simulink model "ProgettoFinaleFSR"  (R2024a)
settings: Solver=VariableStepAuto  StartTime=0.0  StopTime=30  RelTol=1e-3
PreLoadFcn:
  | Ts = 1e-3;
  | m = 1;
InitFcn:
  | %% INITIALIZATION
  | main
  | 
  | %% UAV PARAMETERS
  | 
  | %% SAMPLING TIME
  | Ts=0.001;
  | 
  | %% PLANNER
  | % t_iniz = 0;
  | % ttot=20; %duration
  | % tdead=10; %dead time to evaluate the steady-state
  | % tot_time = ttot + tdead;
  | % t1=linspace(0,ttot,round(ttot/Ts));
  | % t=linspace(0,ttot+tdead,round(ttot/Ts)+round(tdead/Ts));
  | % p= zeros(4,length(t1)); dot_p= zeros(4,length(t1)); ddot_p= zeros(4,length(t1));
  | % p_d= zeros(4,length(t)); dot_p_d= zeros(4,length(t)); ddot_p_d= zeros(4,length(t));
  | % %Initial and final conditions
  | % x0= 0; xf=1; dot_x0= 0; dot_xf=0; ddot_x0=0; ddot_xf=0; dddot_x0 = 0; dddot_xf = 0;
  | % y0= 0; yf=1; dot_y0= 0; dot_yf=0; ddot_y0=0; ddot_yf=0; dddot_y0 = 0; dddot_yf = 0;
  | % z0= -1; zf=-4; dot_z0= 0; dot_zf=0; ddot_z0=0; ddot_zf=0; dddot_z0 = 0; dddot_zf = 0;
  | % psi0 = 0;
  | % psif=deg2rad(20); dot_psi0= 0; dot_psif=0; ddot_psi0=0; ddot_psif=0; dddot_psi0 = 0; dddot_psif = 0;
  | % p0=[x0,y0,z0,psi0]; dot_p0=[dot_x0,dot_y0,dot_z0,dot_psi0]; ddot_p0=[ddot_x0,ddot_y0,ddot_z0,ddot_psi0]; dddot_p0=[dddot_x0,dddot_y0,dddot_z0,dddot_psi0];
  | % pf=[xf,yf,zf,psif]; dot_pf=[dot_xf,dot_yf,dot_zf,dot_psif]; ddot_pf=[ddot_xf,ddot_yf,ddot_zf,ddot_psif]; dddot_pf=[dddot_xf,dddot_yf,dddot_zf,dddot_psif];
  | % %5-th order polynomial
  | % a0=zeros(1,4); a1=zeros(1,4); a2=zeros(1,4); a3=zeros(1,4); a4=zeros(1,4); a5=zeros(1,4); a6 = zeros(1,4); a7 = zeros(1,4);
  | %
  | % for j=1:4
  | %     A = [t_iniz^7, t_iniz^6, t_iniz^5, t_iniz^4, t_iniz^3, t_iniz^2, t_iniz, 1;
  | %         ttot^7, ttot^6, ttot^5, ttot^4, ttot^3, ttot^2, ttot, 1;
  | %         7*t_iniz^6, 6*t_iniz^5, 5*t_iniz^4, 4*t_iniz^3, 3*t_iniz^2, 2*t_iniz, 1, 0;
  | %         7*ttot^6, 6*ttot^5, 5*ttot^4, 4*ttot^3, 3*ttot^2, 2*ttot, 1, 0;
  | %         42*t_iniz^5, 30*t_iniz^4, 20*t_iniz^3, 12*t_iniz^2, 6*t_iniz, 2, 0, 0;
  | %         42*ttot^5, 30*ttot^4, 20*ttot^3, 12*ttot^2, 6*ttot, 2, 0, 0;
  | %         210*t_iniz^4, 120*t_iniz^3, 60*t_iniz^2, 24*t_iniz, 6, 0, 0, 0;
  | %         210*ttot^4, 120*ttot^3, 60*ttot^2, 24*ttot, 6, 0, 0, 0];
  | %     b = [p0(j) pf(j) dot_p0(j) dot_pf(j) ddot_p0(j) ddot_pf(j) dddot_p0(j) dddot_pf(j)]';
  | %     a_temp = A\b;
  | %     a7(j) = a_temp(1);
  | %     a6(j) = a_temp(2);
  | %     a5(j) = a_temp(3);
  | %     a4(j) = a_temp(4);
  | %     a3(j) = a_temp(5);
  | %     a2(j) = a_temp(6);
  | %     a1(j) = a_temp(7);
  | %     a0(j) = a_temp(8);
  | %
  | %     %trajectories
  | %     p(j,:)=a7(j)*t1.^7 + a6(j)*t1.^6 + a5(j)*t1.^5 +a4(j)*t1.^4 +a3(j)*t1.^3 +a2(j)*t1.^2 +a1(j)*t1 +a0(j);
  | %     dot_p(j,:) = 7*a7(j)*t1.^6 + 6*a6(j)*t1.^5 + 5*a5(j)*t1.^4 +4*a4(j)*t1.^3 +3*a3(j)*t1.^2 +2*a2(j)*t1 +a1(j);
  | %     ddot_p(j,:) = 42*a7(j)*t1.^5 + 30*a6(j)*t1.^4 + 5*4*a5(j)*t1.^3 +4*3*a4(j)*t1.^2 +3*2*a3(j)*t1 +2*a2(j);
  | %     %addition of the stead-state terms
  | %     p_d(j,:)=[p(j,:) zeros(1,round(tdead/Ts))+pf(j)];
  | %     dot_p_d(j,:)=[dot_p(j,:) zeros(1,round(tdead/Ts))+dot_pf(j)];
  | %     ddot_p_d(j,:)=[ddot_p(j,:) zeros(1,round(tdead/Ts))+ddot_pf(j)];
  | % end
  | % %data for Simulink
  | % pos_0 = [x0 y0 z0];
  | % lin_vel_0 = [dot_x0 dot_y0 dot_z0];
  | % w_bb_0 = [0 0 0];
  | % csi_d=p_d(1:3,:); dot_csi_d=dot_p_d(1:3,:); ddot_csi_d=ddot_p_d(1:3,:);
  | % psi_d=p_d(4,:); dot_psi_d=dot_p_d(4,:); ddot_psi_d=ddot_p_d(4,:);
values from neighbouring files (symbols this model uses):
  g = 9.81    [main.m]
  intv = [intv,v(i).vec]    [main.m]
  k = ones(r,1)    [gainvalue.m]    (also in main.m = gainvalue(r,a(2:end)))
settings Model: Creator=fabioruggiero  LastModifiedBy=Luca
settings ModelReferenceCC: EnableRefExpFcnMdlSchedulingChecks=on
settings RTWCC: GPUComputeCapability=3.5

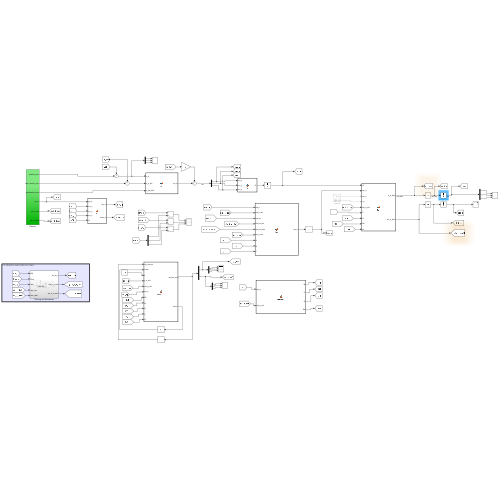
[thumbnail: Simulink's stored preview of the top-level diagram]
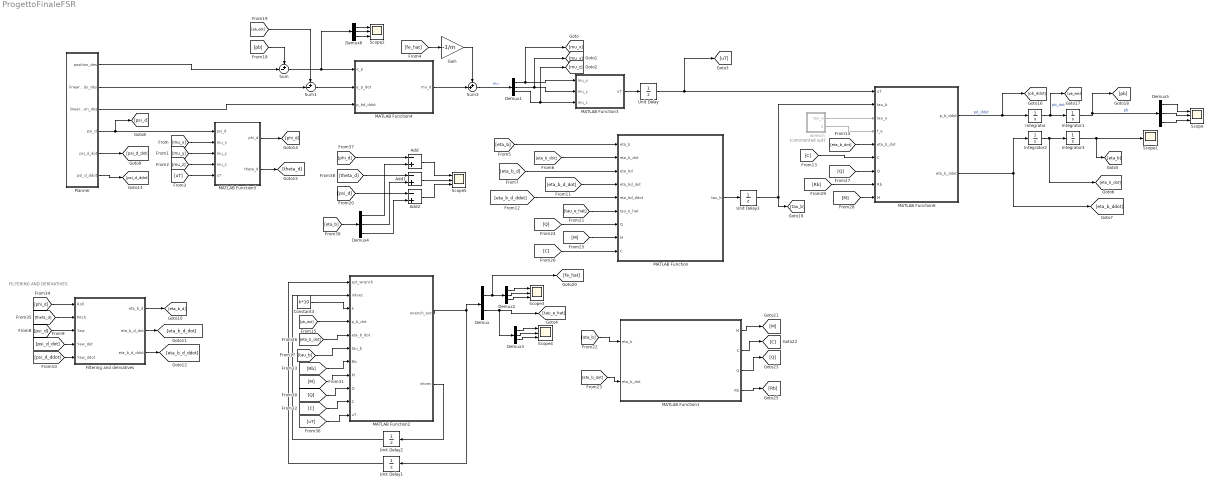
== system ProgettoFinaleFSR ==
  note: FILTERING AND DERIVATIVES
  " wrench" : Subsystem  Commented=on
  Add : Sum  Inputs=-+
  Add1 : Sum  Inputs=-+
  Add2 : Sum  Inputs=-+
  Constant3 : Constant  Value=k*10
  Demux : Demux  Outputs=2
  Demux{1..6} (6 alike) : Demux  Outputs=3
  Filtering and derivatives : Subsystem
  Gain : Gain  Gain=-1/m
  Integrator : Integrator
  Integrator1 : Integrator  InitialCondition=[0; 0; -1]
  Integrator2 : Integrator
  Integrator3 : Integrator
  MATLAB Function : MATLAB Function  TreatAsAtomicUnit=on
  MATLAB Function1 : MATLAB Function  TreatAsAtomicUnit=on
  MATLAB Function2 : MATLAB Function  TreatAsAtomicUnit=on
  MATLAB Function3 : MATLAB Function  TreatAsAtomicUnit=on
  MATLAB Function4 : MATLAB Function  TreatAsAtomicUnit=on
  MATLAB Function5 : MATLAB Function  TreatAsAtomicUnit=on
  MATLAB Function6 : MATLAB Function  TreatAsAtomicUnit=on
  Planner : Subsystem
  Scope{,2..5} (5 alike) : Scope  NumInputPorts=3
  Scope1 : Scope
  Sum : Sum  Inputs=+-|
  Sum1 : Sum  Inputs=+-|
  Sum3 : Sum  Inputs=++|
  Unit Delay : UnitDelay  InitialCondition=m*g  SampleTime=Ts  HasFrameUpgradeWarning=on
  Unit Delay1 : UnitDelay  InitialCondition=zeros(6,1)  SampleTime=Ts  HasFrameUpgradeWarning=on
  Unit Delay2 : UnitDelay  InitialCondition=intv  SampleTime=Ts  HasFrameUpgradeWarning=on
  Unit Delay3 : UnitDelay  SampleTime=Ts  HasFrameUpgradeWarning=on
  wires:
  Planner/2(linear_velocity_des) -> Sum1/2
  MATLAB Function2/2(intvec) -> Unit Delay2/1
  Unit Delay1/1 -> MATLAB Function2/1(est_wrench)
  Constant3/1 -> MATLAB Function2/3(k)
  Unit Delay2/1 -> MATLAB Function2/2("intvec ")
  MATLAB Function2/1(wrench_ext) -> Demux/1, Unit Delay1/1
  Demux1/1 -> [mu_x], MATLAB Function3/1(mu_x)
  Demux1/2 -> [mu_y], MATLAB Function3/2(mu_y)
  Demux1/3 -> [mu_z], MATLAB Function3/3(mu_z)
  Sum/1 -> Demux6/1, MATLAB Function4/1(e_p)
  Integrator1/1 -> Demux5/1, [pb]  "pb"
  Integrator/1 -> [pb_dot], Integrator1/1  "pb_dot"
  MATLAB Function6/1(p_b_ddot) -> [pb_ddot], Integrator/1  "pd_ddot"
  Sum1/1 -> MATLAB Function4/2(e_p_dot)
  Planner/1(position_des) -> Sum/2
  Planner/4(psi_d) -> [psi_d], MATLAB Function5/1(psi_d)
  MATLAB Function5/1(phi_d) -> [phi_d]
  MATLAB Function5/2(theta_d) -> [theta_d]
  [mu_x] -> MATLAB Function5/2(mu_x)
  [mu_y] -> MATLAB Function5/3(mu_y)
  [mu_z] -> MATLAB Function5/4(mu_z)
  [uT] -> MATLAB Function5/5(uT)
  Sum3/1 -> Demux1/1  "mu"
  MATLAB Function4/1(mu_d) -> Sum3/2
  [fe_hat] -> Gain/1
  Integrator2/1 -> [eta_b_dot], Integrator3/1
  Integrator3/1 -> Scope1/1, [eta_b]
  [eta_b] -> MATLAB Function/1(eta_b)
  [eta_b_dot] -> MATLAB Function/2(eta_b_dot)
  [psi_d] -> Filtering and derivatives/3(Yaw)
  [psi_d_ddot] -> Filtering and derivatives/5(Yaw_ddot)
  [theta_d] -> Filtering and derivatives/2(Pitch)
  [phi_d] -> Filtering and derivatives/1(Roll)
  Filtering and derivatives/3(eta_b_d_ddot) -> [eta_b_d_ddot]
  Filtering and derivatives/1(eta_b_d) -> [eta_b_d]
  [psi_d_dot] -> Filtering and derivatives/4(Yaw_dot)
  Filtering and derivatives/2(eta_b_d_dot) -> [eta_b_d_dot]
  Planner/5(psi_d_dot) -> [psi_d_dot]
  Planner/6(psi_d_ddot) -> [psi_d_ddot]
  [eta_b_d] -> MATLAB Function/3(eta_bd)
  [eta_b_d_dot] -> MATLAB Function/4(eta_bd_dot)
  [eta_b_d_ddot] -> MATLAB Function/5(eta_bd_ddot)
  [C] -> MATLAB Function6/6(C)
  [eta_b_dot] -> MATLAB Function6/5(eta_b_dot)
  [eta_b_dot] -> MATLAB Function2/5(eta_b_dot)
  [tau_b] -> MATLAB Function2/6(tau_b)
  [pb] -> Sum/1
  [pb_dot] -> Sum1/1
  Planner/3(linear_acceleration_des) -> MATLAB Function4/3(p_bd_ddot)
  [tau_e_hat] -> MATLAB Function/6(tau_e_hat)
  " wrench"/1(tau_e) -> MATLAB Function6/3(tau_e)
  " wrench"/2(fe_hat) -> MATLAB Function6/4(f_e)
  [eta_b] -> MATLAB Function1/1(eta_b)
  [eta_b_dot] -> MATLAB Function1/2(eta_b_dot)
  MATLAB Function1/1(M) -> [M]
  MATLAB Function1/2(C) -> [C]
  MATLAB Function1/3(Q) -> [Q]
  MATLAB Function1/4(Rb) -> [Rb]
  [Q] -> MATLAB Function/7(Q)
  [M] -> MATLAB Function/8(M)
  [C] -> MATLAB Function/9(C)
  [Q] -> MATLAB Function6/7(Q)
  [M] -> MATLAB Function6/9(M)
  [Rb] -> MATLAB Function6/8(Rb)
  [C] -> MATLAB Function2/10(C)
  [M] -> MATLAB Function2/8(M)
  [Q] -> MATLAB Function2/9(Q)
  [Rb] -> MATLAB Function2/7(Rb)
  [uT] -> MATLAB Function2/11(uT)
  [pb_dot] -> MATLAB Function2/4(p_b_dot)
  MATLAB Function6/2(eta_b_ddot) -> [eta_b_ddot], Integrator2/1
  MATLAB Function3/1(uT) -> Unit Delay/1
  MATLAB Function/1(tau_b) -> Unit Delay3/1
  Unit Delay/1 -> [uT], MATLAB Function6/1(uT)
  Unit Delay3/1 -> MATLAB Function6/2(tau_b), [tau_b]
  Demux2/1 -> Scope3/1
  Demux2/2 -> Scope3/2
  Demux2/3 -> Scope3/3
  Demux/1 -> [fe_hat], Demux2/1
  Demux/2 -> Demux3/1, [tau_e_hat]
  Demux3/3 -> Scope4/3
  Demux3/2 -> Scope4/2
  Demux3/1 -> Scope4/1
  [eta_b] -> Demux4/1
  Add/1 -> Scope5/1
  Add1/1 -> Scope5/2
  Add2/1 -> Scope5/3
  [theta_d] -> Add1/1
  [psi_d] -> Add2/1
  [phi_d] -> Add/1
  Demux4/1 -> Add/2
  Demux4/2 -> Add1/2
  Demux4/3 -> Add2/2
  Demux5/1 -> Scope/1
  Demux5/2 -> Scope/2
  Demux5/3 -> Scope/3
  Demux6/1 -> Scope2/1
  Demux6/2 -> Scope2/2
  Demux6/3 -> Scope2/3
  Gain/1 -> Sum3/1

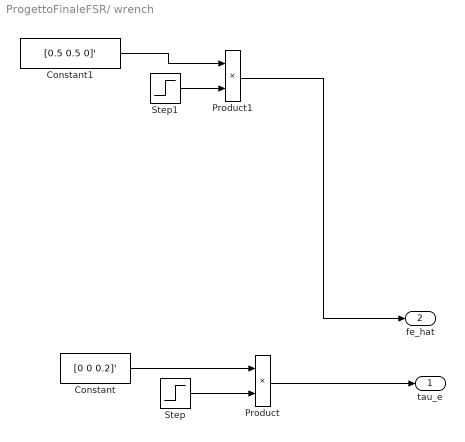
== system ProgettoFinaleFSR/ wrench ==
  Constant : Constant  Value=[0 0 0.2]'
  Constant1 : Constant  Value=[0.5 0.5 0]'
  Product : Product
  Product1 : Product
  Step : Step  Time=10  SampleTime=0
  Step1 : Step  Time=10  SampleTime=0
  tau_e : Outport
  fe_hat : Outport  Port=2
  wires:
  Step1/1 -> Product1/2
  Product/1 -> tau_e/1
  Constant1/1 -> Product1/1
  Constant/1 -> Product/1
  Step/1 -> Product/2
  Product1/1 -> fe_hat/1

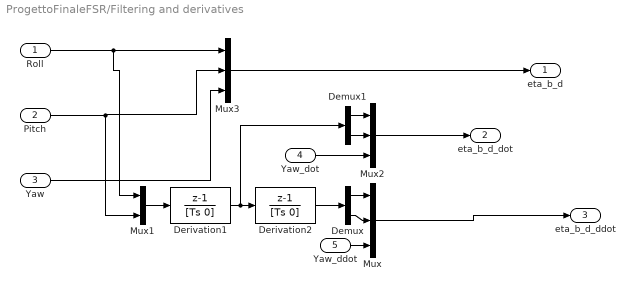
== system ProgettoFinaleFSR/Filtering and derivatives ==
  Roll : Inport
  Pitch : Inport  Port=2
  Yaw : Inport  Port=3
  Yaw_dot : Inport  Port=4
  Yaw_ddot : Inport  Port=5
  Demux : Demux  Outputs=2
  Demux1 : Demux  Outputs=2
  Derivation1 : DiscreteTransferFcn  Numerator=[1 -1]  Denominator=[Ts 0]  InitialStates=[0 0]  SampleTime=Ts
  Derivation2 : DiscreteTransferFcn  Numerator=[1 -1]  Denominator=[Ts 0]  InitialStates=[0 0]  SampleTime=Ts
  Mux : Mux  Inputs=3
  Mux1 : Mux  Inputs=2
  Mux2 : Mux  Inputs=3
  Mux3 : Mux  Inputs=3
  eta_b_d : Outport
  eta_b_d_dot : Outport  Port=2
  eta_b_d_ddot : Outport  Port=3
  wires:
  Derivation1/1 -> Demux1/1, Derivation2/1
  Pitch/1 -> Mux1/2, Mux3/2
  Demux1/1 -> Mux2/1
  Roll/1 -> Mux1/1, Mux3/1
  Mux1/1 -> Derivation1/1
  Demux1/2 -> Mux2/2
  Yaw_dot/1 -> Mux2/3
  Mux3/1 -> eta_b_d/1
  Derivation2/1 -> Demux/1
  Demux/1 -> Mux/1
  Demux/2 -> Mux/2
  Yaw/1 -> Mux3/3
  Mux/1 -> eta_b_d_ddot/1
  Yaw_ddot/1 -> Mux/3
  Mux2/1 -> eta_b_d_dot/1

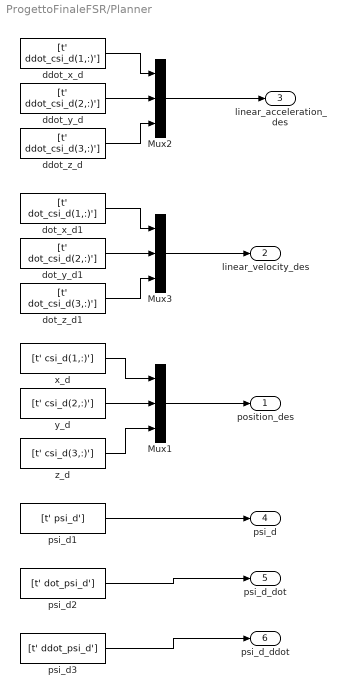
== system ProgettoFinaleFSR/Planner ==
  Mux1 : Mux  Inputs=3
  Mux2 : Mux  Inputs=3
  Mux3 : Mux  Inputs=3
  ddot_x_d : FromWorkspace  VariableName=[t' ddot_csi_d(1,:)']  SampleTime=Ts
  ddot_y_d : FromWorkspace  VariableName=[t' ddot_csi_d(2,:)']  SampleTime=Ts
  ddot_z_d : FromWorkspace  VariableName=[t' ddot_csi_d(3,:)']  SampleTime=Ts
  dot_x_d1 : FromWorkspace  VariableName=[t' dot_csi_d(1,:)']  SampleTime=Ts
  dot_y_d1 : FromWorkspace  VariableName=[t' dot_csi_d(2,:)']  SampleTime=Ts
  dot_z_d1 : FromWorkspace  VariableName=[t' dot_csi_d(3,:)']  SampleTime=Ts
  psi_d1 : FromWorkspace  VariableName=[t' psi_d']  SampleTime=Ts
  psi_d2 : FromWorkspace  VariableName=[t' dot_psi_d']  SampleTime=Ts
  psi_d3 : FromWorkspace  VariableName=[t' ddot_psi_d']  SampleTime=Ts
  x_d : FromWorkspace  VariableName=[t' csi_d(1,:)']  SampleTime=Ts
  y_d : FromWorkspace  VariableName=[t' csi_d(2,:)']  SampleTime=Ts
  z_d : FromWorkspace  VariableName=[t' csi_d(3,:)']  SampleTime=Ts
  position_des : Outport
  linear_velocity_des : Outport  Port=2
  linear_acceleration_des : Outport  Port=3
  psi_d : Outport  Port=4
  psi_d_dot : Outport  Port=5
  psi_d_ddot : Outport  Port=6
  wires:
  y_d/1 -> Mux1/2
  z_d/1 -> Mux1/3
  x_d/1 -> Mux1/1
  ddot_y_d/1 -> Mux2/2
  ddot_z_d/1 -> Mux2/3
  ddot_x_d/1 -> Mux2/1
  Mux2/1 -> linear_acceleration_des/1
  Mux1/1 -> position_des/1
  dot_y_d1/1 -> Mux3/2
  dot_z_d1/1 -> Mux3/3
  dot_x_d1/1 -> Mux3/1
  Mux3/1 -> linear_velocity_des/1
  psi_d1/1 -> psi_d/1
  psi_d2/1 -> psi_d_dot/1
  psi_d3/1 -> psi_d_ddot/1

== matlab function ProgettoFinaleFSR/MATLAB Function4 ==
  data: e_p input; mu_d output; e_p_dot input; p_bd_ddot input
function mu_d = fcn(e_p, e_p_dot, p_bd_ddot)

Kp = 12000*diag([1 1 1]);
Kd = 100*diag([1 1 1]);

mu_d = -Kd*e_p_dot-Kp*e_p+p_bd_ddot;

== matlab function ProgettoFinaleFSR/MATLAB Function5 ==
  data: psi_d input; phi_d output; mu_x input; mu_y input; mu_z input; uT input; theta_d output
function [phi_d,theta_d] = fcn(psi_d,mu_x,mu_y,mu_z,uT)

m = 1;
g = 9.81;


% arg = (m/uT)*(mu_y*cos(psi_d)-mu_x*sin(psi_d));
% 
% if arg < -1
%     phi_d = asin(-1);
% elseif arg > 1
%     phi_d = asin(1);
% else
%     phi_d = asin(arg);
% end

phi_d = asin((m/uT)*(mu_y*cos(psi_d)-mu_x*sin(psi_d)));
theta_d = atan((mu_x*cos(psi_d)+mu_y*sin(psi_d))/(mu_z-g));

== matlab function ProgettoFinaleFSR/MATLAB Function ==
  data: eta_b input; tau_b output; eta_b_dot input; eta_bd input; eta_bd_dot input; eta_bd_ddot input; tau_e_hat input; Q input; M input; C input
function tau_b = fcn(eta_b, eta_b_dot, eta_bd, eta_bd_dot, eta_bd_ddot, tau_e_hat, Q, M, C)

    sigma = 10;
    ni = 10;
    
    Do = 10*diag([1 1 1]);
    Ko = sigma*Do;
    
    e_eta = eta_b - eta_bd;
    e_eta_dot = eta_b_dot - eta_bd_dot;
    v_eta = e_eta_dot + sigma*e_eta;
    eta_r_dot = eta_bd - sigma*e_eta;
    eta_r_ddot = eta_bd_ddot - ni*e_eta_dot;
    
    tau_b = (inv(Q)')*(M*eta_r_ddot+C*eta_r_dot-tau_e_hat-Do*v_eta-Ko*e_eta);

end

== matlab function ProgettoFinaleFSR/MATLAB Function6 ==
  data: uT input; p_b_ddot output; tau_b input; tau_e input; f_e input; eta_b_dot input; C input; eta_b_ddot output; Q input; Rb input; M input
function [p_b_ddot,eta_b_ddot] = fcn(uT,tau_b,tau_e,f_e,eta_b_dot,C,Q,Rb,M)

m = 1;
g = 9.81;
e3 = [0 0 1]';

p_b_ddot = g*e3 - (1/m)*uT*Rb*e3 + f_e;
eta_b_ddot = inv(M)*(-C*eta_b_dot+Q'*tau_b+tau_e);

== matlab function ProgettoFinaleFSR/MATLAB Function2 ==
  data: est_wrench input; intvec input; k input; p_b_dot input size=[3 1]; eta_b_dot input size=[3 1]; tau_b input; wrench_ext output; intvec output; Rb input; M input; Q input; C input; uT input
function [wrench_ext,intvec] = estimation(est_wrench,intvec, k,p_b_dot, eta_b_dot,tau_b,Rb,M,Q,C,uT)

    m = 1;
    g = 9.81;
    e3 = [0 0 1]';
    r = 1;
    
    % Momentum
    q = [m*eye(3) zeros(3) ; zeros(3) M]*[p_b_dot ; eta_b_dot];

    % Integral vector
    intmat= [m*g*e3 - uT*Rb*e3; C'*eta_b_dot + Q' * tau_b];
  
    dt=1e-3;
    gamma=zeros(6,r);

    for i=1:r
        if i==1
            intvec(:,i) = intvec(:,i) + (est_wrench+intmat)*dt;
            gamma(:,i) = k(i)*(q-intvec(:,i));
        else
            intvec(:,i) = intvec(:,i) + (-est_wrench+gamma(:,i-1))*dt;
            gamma(:,i) = k(i)*intvec(:,i);
        end
    end
    wrench_ext = gamma(:,r);

end

== matlab function ProgettoFinaleFSR/MATLAB Function1 ==
  data: eta_b input; M output size=[3 3]; C output size=[3 3]; Q output size=[3 3]; Rb output size=[3 3]; eta_b_dot input
function [M,C,Q,Rb] = matrices(eta_b,eta_b_dot)

Ib = diag([1.2416 1.2416 2*1.2416]);


phi = eta_b(1);
theta = eta_b(2);
psi = eta_b(3);


phi_dot = eta_b_dot(1);
theta_dot = eta_b_dot(2);
psi_dot = eta_b_dot(3);

% Q matrix
Q =[1 0 -sin(theta); 
      0 cos(phi) cos(theta)*sin(phi); 
      0 -sin(phi) cos(theta)*cos(phi)];


Q_dot=[0 0 -theta_dot*cos(theta); 
          0 -phi_dot*sin(phi) (theta_dot*-sin(theta)*sin(phi))+(cos(theta)*phi_dot*cos(phi)); 
          0 phi_dot*-cos(phi) (theta_dot*-sin(theta)*cos(phi))+(cos(theta)*phi_dot*-sin(phi))];

% M matrix
M = zeros(3,3);
M = (Q')*Ib*Q;

% C matrix
C = Q'*skew(Q*eta_b_dot)*Ib*Q+Q'*Ib*Q_dot;

% Rb matrix
Rb = [cos(theta)*cos(psi) sin(phi)*sin(theta)*cos(psi)-cos(phi)*sin(psi) cos(phi)*sin(theta)*cos(psi)+sin(phi)*sin(psi);
      cos(theta)*sin(psi) sin(phi)*sin(theta)*sin(psi)+cos(phi)*cos(psi) cos(phi)*sin(theta)*sin(psi)-sin(phi)*cos(psi);
      -sin(theta) sin(phi)*cos(theta) cos(phi)*cos(theta)];

function S = skew(v)
    if(numel(v)~= 1)
        S= [0 -v(3) v(2); 
            v(3) 0 -v(1);
            -v(2) v(1) 0];
    else
        S= zeros(3);
    end
end

end

== matlab function ProgettoFinaleFSR/MATLAB Function3 ==
  data: mu_x input; uT output; mu_y input; mu_z input
function uT = fcn(mu_x,mu_y,mu_z)

m = 1;
g = 9.81;

uT = m*sqrt(mu_x^2+mu_y^2+(mu_z^2-g)^2);
